simulink model "motore"  (R2022a)
settings: Solver=ode45  StartTime=0.0  StopTime=5  MaxStep=0.0001  RelTol=1e-3
values from neighbouring files (symbols this model uses):
  d = 1 / sqrt(2)    [ex1.m]    (also in ex2.m)
  Kp = kc / 4    [ex2.m]    (also in ex3.m = 0.744)
  rads2rpm = 60 / (2 * pi)    (= 9.54929658551)    [ex2.m]    (also in ex3.m)
  w = step(Ww, t, w1)    [ex2.m]
  w0 = 0    [ex3.m]
undefined symbols (not defined in the file or in its folder): diff, mot
settings Model: Creator=loren  LastModifiedBy=loren
settings DataIOCC: ReturnWorkspaceOutputs=off

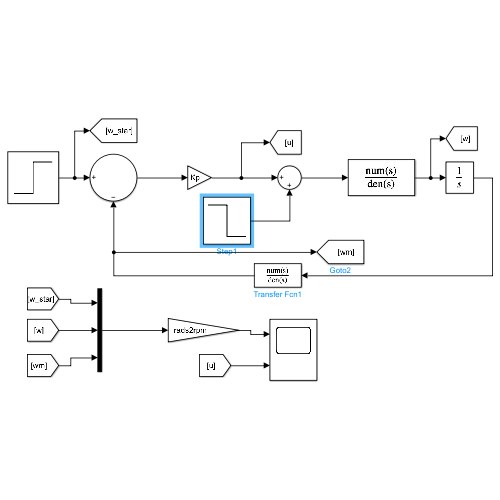
[thumbnail: Simulink's stored preview of the top-level diagram]
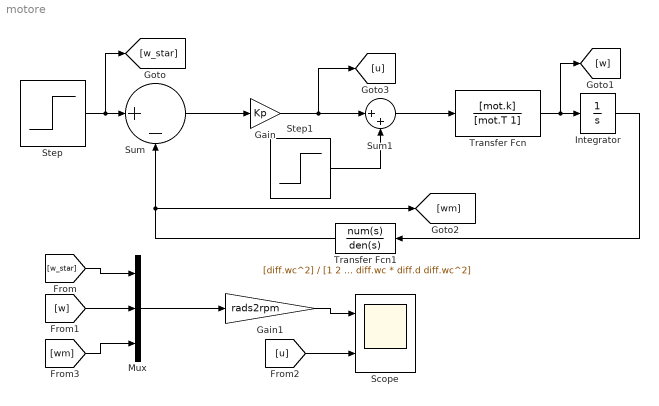
== system motore ==
  Gain : Gain  Gain=Kp
  Gain1 : Gain  Gain=rads2rpm
  Integrator : Integrator  InitialCondition=w0
  Mux : Mux  Inputs=3
  Scope : Scope  NumInputPorts=2
  Step : Step  Time=w.t  After=w.A  SampleTime=0
  Step1 : Step  Time=d.t  After=d.A  SampleTime=0
  Sum : Sum  Inputs=|+-
  Sum1 : Sum  Inputs=|++
  Transfer Fcn : TransferFcn  Numerator=[mot.k]  Denominator=[mot.T 1]
  Transfer Fcn1 : TransferFcn  Numerator=[diff.wc^2]  Denominator=[1 2 * diff.wc * diff.d diff.wc^2]
  wires:
  [u] -> Scope/2
  [wm] -> Mux/3
  Gain/1 -> [u], Sum1/1
  Transfer Fcn/1 -> [w], Integrator/1
  Gain1/1 -> Scope/1
  Step/1 -> [w_star], Sum/1
  Sum1/1 -> Transfer Fcn/1
  Mux/1 -> Gain1/1
  [w] -> Mux/2
  [w_star] -> Mux/1
  Sum/1 -> Gain/1
  Integrator/1 -> Transfer Fcn1/1
  Step1/1 -> Sum1/2
  Transfer Fcn1/1 -> Sum/2, [wm]
